simulink model "pendule"  (Simulink 6.1)
settings: Solver=ode45  StartTime=0.0  StopTime=10  MaxStep=10  RelTol=1e-3  AbsTol=1e-3
settings Model: LastModifiedBy=bengaidm  ExtModeTrigMode=oneshot  ExtModeArmWhenConnect=off
settings DataIOCC: LimitDataPoints=off  SaveOutput=off  SaveTime=off
settings OptimizationCC: BlockReduction=off  BooleanDataType=off
settings HardwareCC: TargetUnknown=on

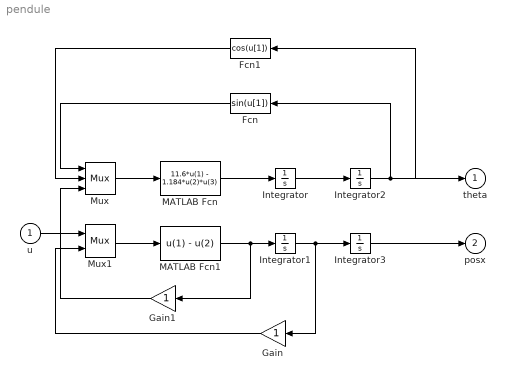
== system pendule ==
  u : Inport  Port=1  LatchInput=off
  Fcn : Fcn  Orientation=left
  Fcn1 : Fcn  Orientation=left  Expr=cos(u[1])
  Gain : Gain  Orientation=left  SaturateOnIntegerOverflow=on
  Gain1 : Gain  Orientation=left  SaturateOnIntegerOverflow=on
  Integrator{,1..3} (4 alike) : Integrator
  MATLAB Fcn : MATLABFcn  MATLABFcn=11.6*u(1) - 1.184*u(2)*u(3)  OutputDimensions=1
  MATLAB Fcn1 : MATLABFcn  MATLABFcn=u(1) - u(2)  OutputDimensions=1
  Mux : Mux  Inputs=3
  Mux1 : Mux  Inputs=2
  theta : Outport
  posx : Outport  Port=2
  wires:
  u/1 -> Mux1/1
  Gain/1 -> Mux1/2
  Gain1/1 -> Mux/3
  MATLAB Fcn1/1 -> Gain1/1, Integrator1/1
  MATLAB Fcn/1 -> Integrator/1
  Mux/1 -> MATLAB Fcn/1
  Mux1/1 -> MATLAB Fcn1/1
  Fcn1/1 -> Mux/2
  Fcn/1 -> Mux/1
  Integrator2/1 -> Fcn1/1, Fcn/1, theta/1
  Integrator1/1 -> Gain/1, Integrator3/1
  Integrator/1 -> Integrator2/1
  Integrator3/1 -> posx/1
